simulink model "cep51"  (R2021a)
settings: Solver=VariableStepAuto  StartTime=0.0  StopTime=20000  RelTol=1e-3
values from neighbouring files (symbols this model uses):
  Ts = 0.5    [Distillation_Column_model_identification.m]    (also in Distillation_Column_model_variance.m; fourvary.m = 8)
libraries: cstblocks x1, dspsrcs4 x1
settings Model: Creator=dell  LastModifiedBy=dell
settings DataIOCC: LoadExternalInput=on

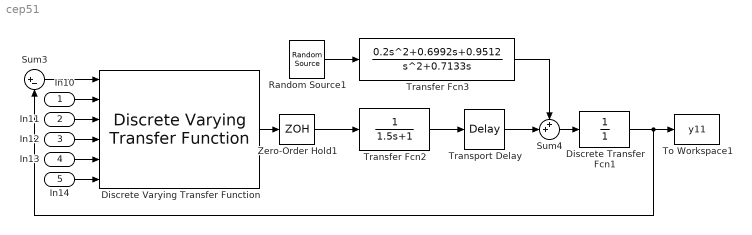
== system cep51 ==
  In10 : Inport
  In11 : Inport  Port=2
  In12 : Inport  Port=3
  In13 : Inport  Port=4
  In14 : Inport  Port=5
  Discrete Transfer Fcn1 : DiscreteTransferFcn  Denominator=[1]  SampleTime=Ts
      mask Display: disp('sampler')
  Discrete Varying Transfer Function : cstblocks/Linear Parameter Varying/Discrete Varying Transfer Function  N=2  Ts=-1
      settings: SourceProductBaseCode=CT
  Random Source1 : dspsrcs4/Random Source  SrcType=Gaussian  NormMethod=Ziggurat  CltLength=12  MinVal=-1  MaxVal=1  MeanVal=0  VarVal=1  RepMode=Specify seed  rawSeed=1  IsInherit=off  SampMode=Continuous  SampTime=1  SampFrame=1  DataType=Double  OutComplex=Real  OutputFrames=off
  Sum3 : Sum  Inputs=|+-
  Sum4 : Sum  Inputs=++|
  To Workspace1 : ToWorkspace  VariableName=y11  SampleTime=Ts
  Transfer Fcn2 : TransferFcn  Denominator=[1.5 1]
  Transfer Fcn3 : TransferFcn  Numerator=[0.2 0.6992 0.9512]  Denominator=[1 0.7133 0]
  Transport Delay : TransportDelay  DelayTime=5
  Zero-Order Hold1 : ZeroOrderHold  SampleTime=Ts
  wires:
  Discrete Varying Transfer Function/1 -> Zero-Order Hold1/1
  Discrete Transfer Fcn1/1 -> To Workspace1/1, Sum3/2
  Sum4/1 -> Discrete Transfer Fcn1/1
  Transfer Fcn3/1 -> Sum4/1
  Random Source1/1 -> Transfer Fcn3/1
  Transport Delay/1 -> Sum4/2
  Transfer Fcn2/1 -> Transport Delay/1
  Zero-Order Hold1/1 -> Transfer Fcn2/1
  In10/1 -> Discrete Varying Transfer Function/2
  In11/1 -> Discrete Varying Transfer Function/3
  In12/1 -> Discrete Varying Transfer Function/4
  In13/1 -> Discrete Varying Transfer Function/5
  In14/1 -> Discrete Varying Transfer Function/6
  Sum3/1 -> Discrete Varying Transfer Function/1
